simulink model "Control_PID"  (R2017b)
settings: Solver=FixedStepAuto  StartTime=0.0  StopTime=inf  RelTol=1e-3  EnableMultiTasking=on
InitFcn:
  | TuneGain = 1
undefined symbols (not defined in the file): armar, gas, kk1, kk2
libraries: pixhawk_slib_sensors_actuators x2, simulink x1
Description:
  | PX4 PSP Demo Model - parameter tune model
  | 
  | tuning parameters in external mode example
settings Model: SimulationMode=external  ExtModeBatchMode=on  TunableVars=armar,gas,kk1,kk2,kk3  TunableVarsStorageClass=Auto,Auto,Auto,Auto,Auto  TunableVarsTypeQualifier=,,,,  Creator=skuznick  LastModifiedBy=CPOH
settings DataIOCC: LimitDataPoints=on  SaveFormat=Array  SignalLoggingSaveFormat=ModelDataLogs
settings OptimizationCC: DefaultParameterBehavior=Inlined  LifeSpan=1  MaxStackSize=64
settings DebuggingCC: SolverPrmCheckMsg=warning  MultiTaskDSMMsg=warning  MultiTaskCondExecSysMsg=none  AllowSymbolicDim=off  SFUnexpectedBacktrackingDiag=warning  SFNoUnconditionalDefaultTransitionDiag=warning  SFExecutionAtInitializationDiag=none
settings HardwareCC: ProdBitPerPointer=32  ProdBitPerSizeT=32  ProdBitPerPtrDiffT=32  ProdLargestAtomicInteger=Long  ProdLargestAtomicFloat=Double  ProdIntDivRoundTo=Undefined  ProdWordSize=32  ProdHWDeviceType=ARM Compatible->ARM Cortex
settings ModelReferenceCC: PropagateSignalLabelsOutOfModel=off
settings SFSimCC: MATLABDynamicMemAlloc=off
settings RTWCC: SystemTargetFile=ert.tlc  HardwareBoard=Pixhawk PX4  TLCOptions=-aInlineSetEventsForThisBaseRateFcn=TLC_FALSE -aSuppressMultiTaskScheduler=TLC_FALSE -aRateBasedStepFcn=0  TemplateMakefile=ert_default_tmf  GenerateReport=on  Toolchain=Pixhawk Toolchain  IncludeHyperlinkInReport=on  LaunchReport=on  GenerateTraceInfo=on  GenerateTraceReport=on  GenerateTraceReportSl=on  GenerateTraceReportSf=on  GenerateTraceReportEml=on  GenerateCodeMetricsReport=on
settings CodeAppCC: IgnoreCustomStorageClasses=off  StateflowObjectComments=on
settings ERTTargetCC: MultiwordLength=2048  ExtMode=on  ExtModeTransport=1  ExtModeStaticAllocSize=10000  ExtModeMexFile=ext_serial_win32_comm  ExtModeMexArgs=1 4 115200  ERTCustomFileTemplate=px4_codertarget_file_process.tlc  ConvertIfToSwitch=off  SuppressUnreachableDefaultCases=off
settings ConfigComp: CovMetricSettings=dw  CovHtmlReporting=on  CovSaveCumulativeToWorkspaceVar=on  CovSaveSingleToWorkspaceVar=on  CovExternalEMLEnable=off  CovSFcnEnable=off

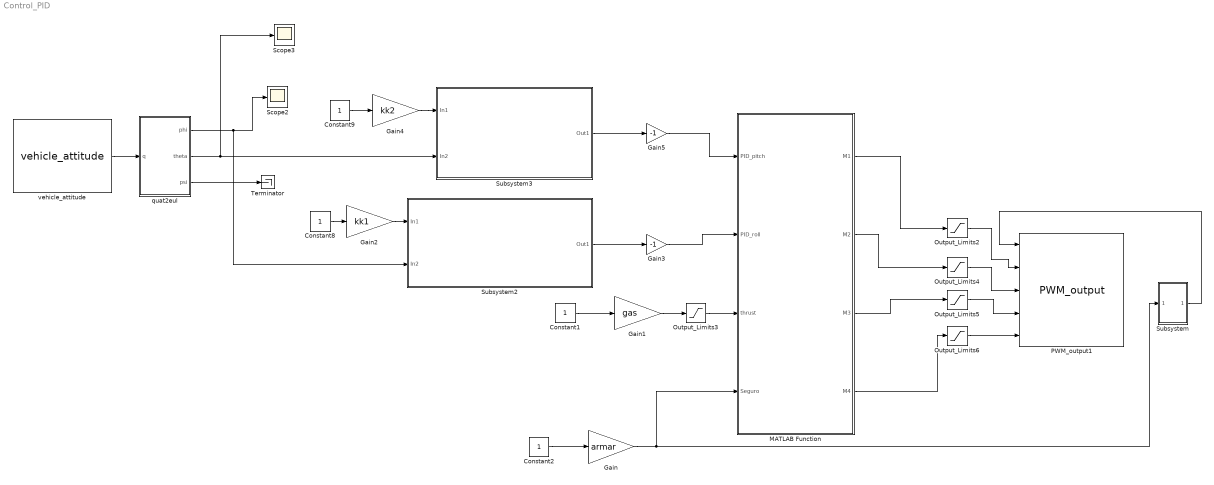
== system Control_PID ==
  Constant{1..2,8..9} (4 alike) : Constant  OutDataTypeStr=single
  Gain : Gain  Gain=armar
  Gain1 : Gain  Gain=gas
  Gain2 : Gain  Gain=kk1
  Gain3 : Gain  Gain=-1
  Gain4 : Gain  Gain=kk2
  Gain5 : Gain  Gain=-1
  MATLAB Function : MATLAB Function  TreatAsAtomicUnit=on
  Output_Limits{2,4..6} (4 alike) : Saturate  UpperLimit=1500  LowerLimit=1000
  Output_Limits3 : Saturate  UpperLimit=30  LowerLimit=0
  PWM_output1 : pixhawk_slib_sensors_actuators/PWM_output  pub_outputs=on  pwm_rate=400Hz  show_pwm1=on  show_pwm5=off  show_pwm2=on  show_pwm6=off  show_pwm3=on  show_pwm7=off  show_pwm4=on  show_pwm8=off
      settings: SourceProductName=Pixhawk Target Blocks
  Scope2 : Scope
  Scope3 : Scope
  Subsystem : Subsystem
  Subsystem2 : Subsystem
  Subsystem3 : Subsystem
  Terminator : Terminator
  quat2eul : MATLAB Function  TreatAsAtomicUnit=on
  vehicle_attitude : pixhawk_slib_sensors_actuators/vehicle_attitude  sampletime=0.004  show_r=off  show_p=off  show_y=off  show_q=on  show_ts=off
      settings: SourceProductName=Pixhawk Target Blocks
  wires:
  Output_Limits5/1 -> PWM_output1/4
  Output_Limits4/1 -> PWM_output1/3
  Gain/1 -> MATLAB Function/4(Seguro), Subsystem/1(In1)
  Output_Limits6/1 -> PWM_output1/5
  MATLAB Function/2(M2) -> Output_Limits4/1
  MATLAB Function/4(M4) -> Output_Limits6/1
  MATLAB Function/1(M1) -> Output_Limits2/1
  MATLAB Function/3(M3) -> Output_Limits5/1
  Output_Limits2/1 -> PWM_output1/2
  Constant1/1 -> Gain1/1
  vehicle_attitude/1 -> quat2eul/1(q)
  Gain1/1 -> Output_Limits3/1
  Constant2/1 -> Gain/1
  Constant8/1 -> Gain2/1
  Subsystem/1(Out1) -> PWM_output1/1
  Output_Limits3/1 -> MATLAB Function/3(thrust)
  quat2eul/1(phi) -> Scope2/1, Subsystem2/2(In2)
  Gain3/1 -> MATLAB Function/2(PID_roll)
  Subsystem2/1(Out1) -> Gain3/1
  Gain2/1 -> Subsystem2/1(In1)
  quat2eul/2(theta) -> Scope3/1, Subsystem3/2(In2)
  Constant9/1 -> Gain4/1
  Gain5/1 -> MATLAB Function/1(PID_pitch)
  Subsystem3/1(Out1) -> Gain5/1
  Gain4/1 -> Subsystem3/1(In1)
  quat2eul/3(psi) -> Terminator/1

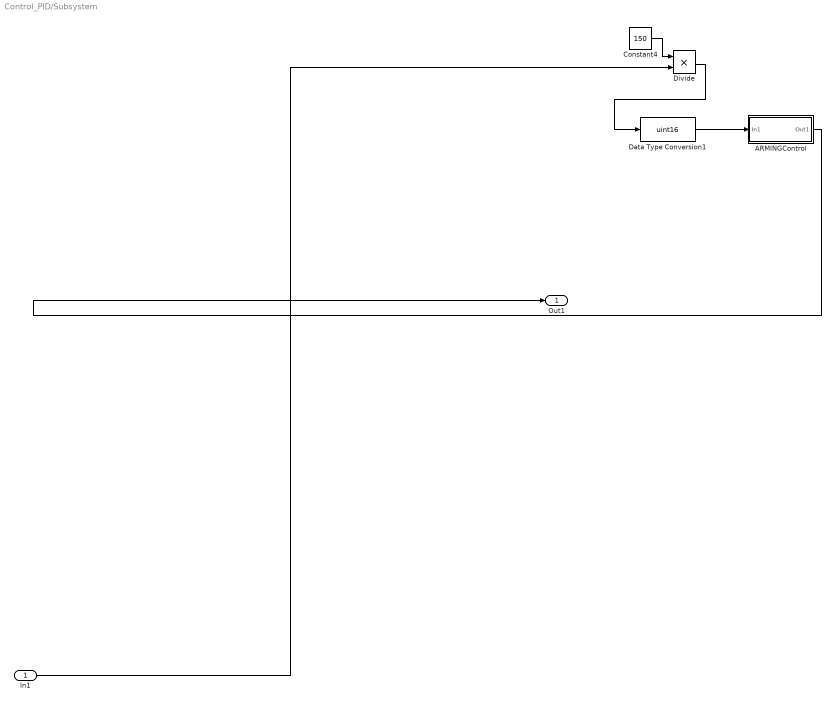
== system Control_PID/Subsystem ==
  In1 : Inport
  ARMINGControl : Subsystem
  Constant4 : Constant  Value=150  OutDataTypeStr=uint16
  Data Type Conversion1 : DataTypeConversion  OutDataTypeStr=uint16
  Divide : Product  Inputs=**
  Out1 : Outport
  wires:
  In1/1 -> Divide/2
  Constant4/1 -> Divide/1
  Data Type Conversion1/1 -> ARMINGControl/1(In1)
  ARMINGControl/1(Out1) -> Out1/1
  Divide/1 -> Data Type Conversion1/1

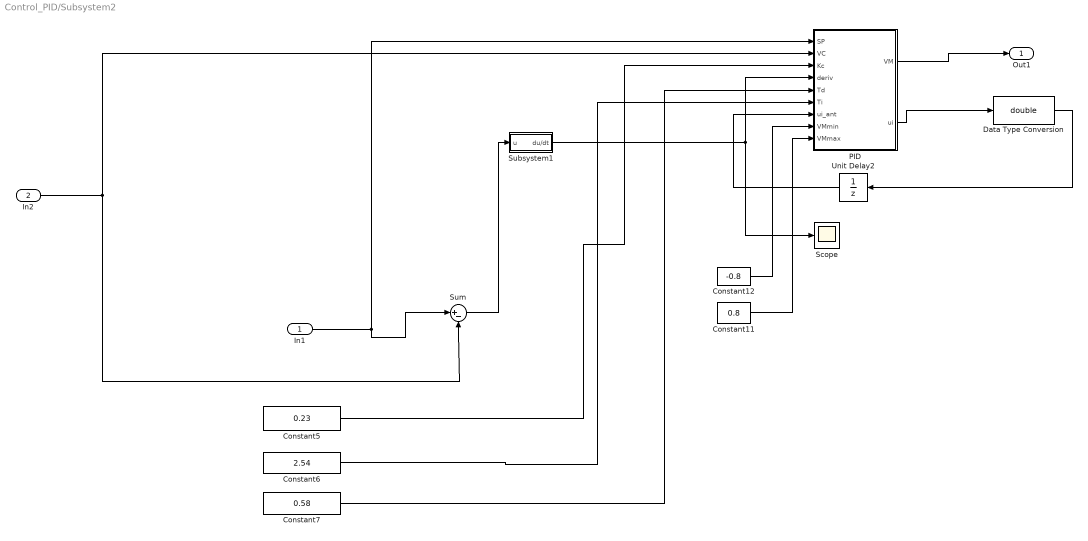
== system Control_PID/Subsystem2 ==
  In1 : Inport
  In2 : Inport  Port=2
  Constant11 : Constant  Value=0.8  OutDataTypeStr=single
  Constant12 : Constant  Value=-0.8  OutDataTypeStr=single
  Constant5 : Constant  Value=0.23  OutDataTypeStr=single
  Constant6 : Constant  Value=2.54  OutDataTypeStr=single
  Constant7 : Constant  Value=0.58  OutDataTypeStr=single
  Data Type Conversion : DataTypeConversion  OutDataTypeStr=double
  PID : MATLAB Function  TreatAsAtomicUnit=on
  Scope : Scope
  Subsystem1 : Subsystem
  Sum : Sum  Inputs=|+-
  Unit Delay2 : UnitDelay  SampleTime=-1
  Out1 : Outport
  wires:
  In2/1 -> Sum/2, PID/2(VC)
  PID/1(VM) -> Out1/1
  Sum/1 -> Subsystem1/1(u)
  Constant6/1 -> PID/6(Ti)
  Subsystem1/1(du/dt) -> Scope/1, PID/4(deriv)
  Unit Delay2/1 -> PID/7(ui_ant)
  Constant11/1 -> PID/9(VMmax)
  In1/1 -> Sum/1, PID/1(SP)
  Constant7/1 -> PID/5(Td)
  Data Type Conversion/1 -> Unit Delay2/1
  Constant12/1 -> PID/8(VMmin)
  Constant5/1 -> PID/3(Kc)
  PID/2(ui) -> Data Type Conversion/1

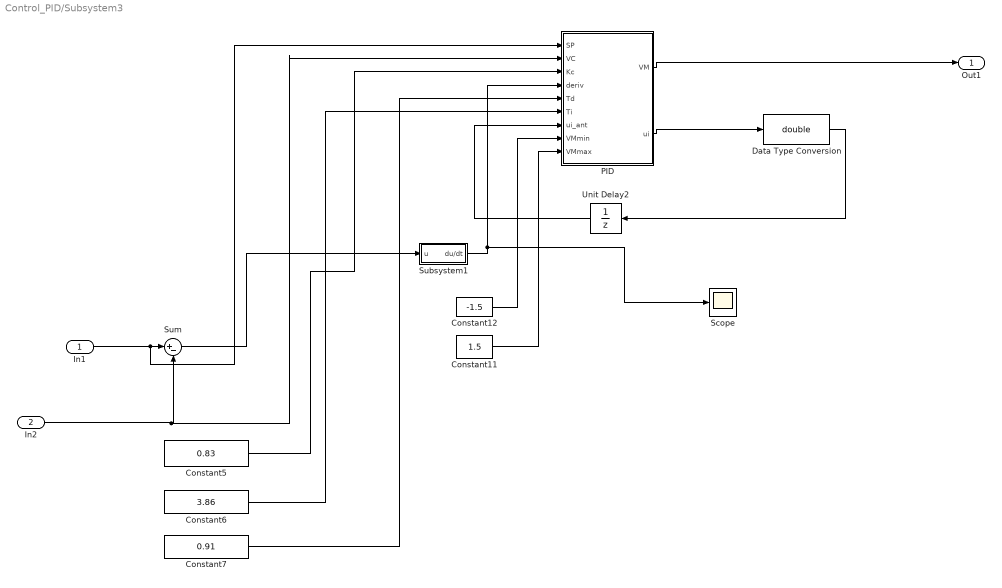
== system Control_PID/Subsystem3 ==
  In1 : Inport
  In2 : Inport  Port=2
  Constant11 : Constant  Value=1.5  OutDataTypeStr=single
  Constant12 : Constant  Value=-1.5  OutDataTypeStr=single
  Constant5 : Constant  Value=0.83  OutDataTypeStr=single
  Constant6 : Constant  Value=3.86  OutDataTypeStr=single
  Constant7 : Constant  Value=0.91  OutDataTypeStr=single
  Data Type Conversion : DataTypeConversion  OutDataTypeStr=double
  PID : MATLAB Function  TreatAsAtomicUnit=on
  Scope : Scope
  Subsystem1 : Subsystem
  Sum : Sum  Inputs=|+-
  Unit Delay2 : UnitDelay  SampleTime=-1
  Out1 : Outport
  wires:
  In2/1 -> PID/2(VC), Sum/2
  Constant6/1 -> PID/6(Ti)
  Sum/1 -> Subsystem1/1(u)
  Subsystem1/1(du/dt) -> Scope/1, PID/4(deriv)
  Data Type Conversion/1 -> Unit Delay2/1
  Constant5/1 -> PID/3(Kc)
  Constant11/1 -> PID/9(VMmax)
  Unit Delay2/1 -> PID/7(ui_ant)
  PID/1(VM) -> Out1/1
  PID/2(ui) -> Data Type Conversion/1
  Constant7/1 -> PID/5(Td)
  In1/1 -> PID/1(SP), Sum/1
  Constant12/1 -> PID/8(VMmin)

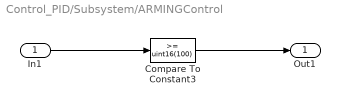
== system Control_PID/Subsystem/ARMINGControl ==
  In1 : Inport
  Compare To Constant3 : simulink/Logic and Bit Operations/Compare To Constant  relop=>=  const=uint16(100)  OutDataTypeStr=boolean
  Out1 : Outport
  wires:
  Compare To Constant3/1 -> Out1/1
  In1/1 -> Compare To Constant3/1

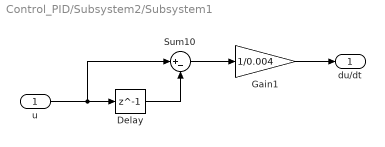
== system Control_PID/Subsystem2/Subsystem1 ==
  u : Inport
  Delay : Delay  DelayLength=1  InitialCondition=0
  Gain1 : Gain  Gain=1/0.004
  Sum10 : Sum  Inputs=|+-
  du/dt : Outport
  wires:
  Gain1/1 -> du/dt/1
  Sum10/1 -> Gain1/1
  Delay/1 -> Sum10/2
  u/1 -> Delay/1, Sum10/1

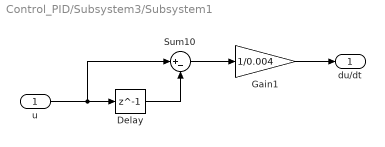
== system Control_PID/Subsystem3/Subsystem1 ==
  u : Inport
  Delay : Delay  DelayLength=1  InitialCondition=0
  Gain1 : Gain  Gain=1/0.004
  Sum10 : Sum  Inputs=|+-
  du/dt : Outport
  wires:
  Gain1/1 -> du/dt/1
  Sum10/1 -> Gain1/1
  Delay/1 -> Sum10/2
  u/1 -> Delay/1, Sum10/1

== matlab function Control_PID/MATLAB Function ==
  data: PID_pitch input; PID_roll input; M1 output; M2 output; M3 output; M4 output; thrust input; Seguro input
function [M1,M2,M3,M4] = fcn(PID_pitch,PID_roll,thrust,Seguro)




k_psi1=0;  %con integrador
k_psi2=0;  %con integrador



ke_psi=0;


db=0.0912; %Diagonal de motor al cento= 129 mm
nb=0.25; %4 brazos = 1/4  %Fuerza entre 4

%Coeficientes funcion PWM-thrust motor a*x^2+b*x+c
a=0.0452;
b=21.649;
%c=2.86;
c=0;

pitch=0;
roll=0;
yaw=0;


ke_psi=0;
e_psi=0;

pitch=PID_pitch;
roll=PID_roll;
yaw=PID_yaw;


%Torque entre 4 motores (entre 4, entre 2 =1/8)

pitch=pitch*nb/db; 
roll=roll*nb/db;
yaw=yaw*nb/db;

pitch=a*pitch^2+b*pitch+c;
roll=a*roll^2+b*roll+c;
yaw=a*yaw^2+b*yaw+c;

pitch=-pitch;
roll=-roll;
yaw=-yaw;
%inhabilitar yaw

%roll=0;
yaw=0;
%pitch=0;

% MIXER MOTORES -------------------------------------------------
idle_PWM = uint16(1000);

M1=uint16((roll+pitch-yaw+thrust)*10)+idle_PWM;
M2=uint16((-roll+pitch+yaw+thrust)*10)+idle_PWM;
M3=uint16((-roll-pitch-yaw+thrust)*10)+idle_PWM;
M4=uint16((roll-pitch+yaw+thrust)*10)+idle_PWM;



if Seguro==0
   M1=idle_PWM;
   M2=idle_PWM;
   M3=idle_PWM;
   M4=idle_PWM;
end

== matlab function Control_PID/Subsystem3/PID ==
  data: SP input; VM output; VC input; Kc input; deriv input; Td input; Ti input; ui_ant input; ui output; VMmin input; VMmax input
function [VM,ui] = fcn(SP,VC,Kc,deriv,Td,Ti,ui_ant,VMmin,VMmax)
  
e=SP-VC;

up=Kc*e;

ud=Kc*Td*deriv;

Ts=0.004;

e=SP-VC;

ki=(Kc*Ts)/Ti;

kie=ki*e;

ui=ui_ant+kie;

 VM=up+ui+ud;

 
if (VM<VMmin)
      VM=VMmin;
   
  ui=single(ui_ant);
 end
 if (VM>VMmax)
      VM=VMmax;
      ui=single(ui_ant);
 end

== matlab function Control_PID/Subsystem2/PID ==
  data: SP input; VM output; VC input; Kc input; deriv input; Td input; Ti input; ui_ant input; ui output; VMmin input; VMmax input
function [VM,ui] = fcn(SP,VC,Kc,deriv,Td,Ti,ui_ant,VMmin,VMmax)
  
e=SP-VC;

up=Kc*e;

ud=Kc*Td*deriv;

Ts=0.004;

e=SP-VC;

ki=(Kc*Ts)/Ti;

kie=ki*e;

ui=ui_ant+kie;

 VM=up+ui+ud;


if (VM<VMmin)
      VM=VMmin;
   
  ui=single(ui_ant);
 end
 if (VM>VMmax)
      VM=VMmax;
         
        ui=single(ui_ant);
 end

== matlab function Control_PID/quat2eul ==
  data: q input; phi output; theta output; psi output
function [phi,theta,psi] = quat2eul(q)
% Conversion from Quaternion to Euler angles based on the PX4 Firmware
% v1.6.5 release.
% 
% Quaternion -> DCM -> Euler Angles
% INPUT:
%   q: Quaternion vector of the format: (a + bi + cj + dk)
% OUTPUT:
%   [phi,theta,psi]: Euler angles in radians.
% 
 
    a = q(1);
    b = q(2);
    c = q(3);
    d = q(4);

    aSq = a*a;
    bSq = b*b;
    cSq = c*c;
    dSq = d*d;

    d_pi2 = pi/2;

    % quaternion_to_dcm
    dcm00 = aSq + bSq - cSq - dSq;
    % dcm01 = 2*(b*c - a*d);
    dcm02 = 2*(a*c + b*d);
    dcm10 = 2*(b*c + a*d);
    % dcm11 = aSq - bSq + cSq - dSq;
    dcm12 = 2*(c*d - a*b);
    dcm20 = 2*(b*d - a*c);
    dcm21 = 2*(a*b + c*d);
    dcm22 = aSq - bSq - cSq + dSq;

    % dcm_to_euler
    theta = asin(-dcm20);
    if abs(theta - d_pi2) < 1.0e-3
        phi = single(0.0);
        psi = atan2(dcm12, dcm02);
    elseif abs(theta + d_pi2) < 1.0e-3
        phi = single(0.0);
        psi = atan2(-dcm12, -dcm02);
    else
        phi = atan2(dcm21, dcm22);
        psi = atan2(dcm10, dcm00);
    end

end
